simulink model "YouTubeVideo_IK_wp"  (R2023b)
settings: Solver=VariableStepAuto  StartTime=0.0  StopTime=6  RelTol=1e-3
values from neighbouring files (symbols this model uses):
  m = d(6)*ay-py    [niyundongxue.m]
undefined symbols (not defined in the file or in its folder): a1, a2, a3, d1, d4, fc1, fc2, fc3, fc4, fc5, fc6, fv1, fv2, fv3, fv4, fv5, fv6, Ia1, Ia2, Ia3, Ia4, Ia5, Ia6, Ic111, Ic112, Ic113, Ic122, Ic123, Ic133, Ic211, Ic212, Ic213, Ic222, Ic223, Ic233, Ic311, Ic312, Ic313, Ic322, Ic323, Ic333, Ic411, Ic412, Ic413, Ic422, Ic423, Ic433, Ic511, Ic512, Ic513, Ic522, Ic523, Ic533, Ic611, Ic612, Ic613, Ic622, Ic623, Ic633, Levenberg ... (+28)
libraries: sm_lib x56, nesl_utility x31, robotcorelib x3, robotmaniplib x2, simulink x2
(part 2 of 2)

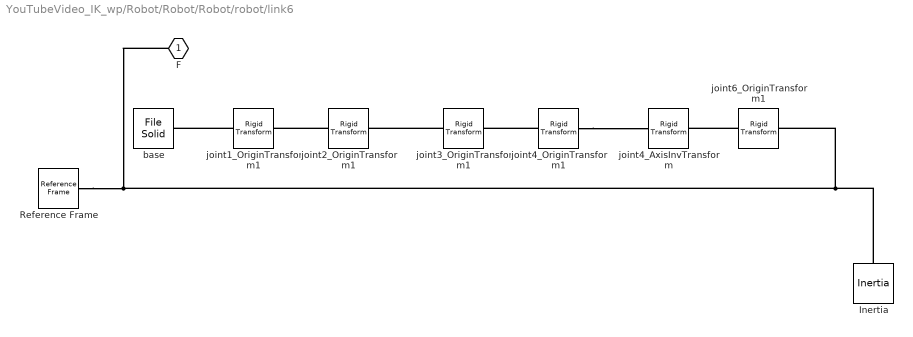
== system YouTubeVideo_IK_wp/Robot/Robot/Robot/robot/link6 ==
  Inertia : sm_lib/Body Elements/Inertia  InertiaType=Custom  Mass=m6  MassUnits=kg  CenterOfMass=[mc61 mc62 mc63]  CenterOfMassUnits=m  MomentsOfInertia=[Ic611 Ic622 Ic633 ]  MomentsOfInertiaUnits=kg*m^2  ProductsOfInertia=[Ic623 Ic613 Ic612]  ProductsOfInertiaUnits=kg*m^2  GraphicType=Marker  MarkerShape=Inertia  MarkerSize=20  GraphicVisPropType=SimpleVisualProperties  GraphicDiffuseColor=[0.5 0.5 0.5]  GraphicSpecularColor=[0.5 0.5 0.5 1.0]  GraphicAmbientColor=[0.15 0.15 0.15 1.0]  GraphicEmissiveColor=[0.0 0.0 0.0 1.0]  GraphicShininess=75  GraphicOpacity=1.0
  Reference Frame : sm_lib/Frames and Transforms/Reference Frame
  base : sm_lib/Body Elements/File Solid  ExtGeomFileName=/home/jiehuang/Documents/Custom-Robot/Matlab_Study/Matlab2023Project/IntroductionBook/程序/XB4模型/XB4-6.STL  UnitType=Custom  ExtGeomFileUnits=mm  StepReaderType=HEX  ExportConvexHullGeometry=off  InertiaType=Custom  Mass=0  MassUnits=kg  CenterOfMass=[0 0 0]  CenterOfMassUnits=m  MomentsOfInertia=[0 0 0]  MomentsOfInertiaUnits=kg*m^2  ProductsOfInertia=[0 0 0]  ProductsOfInertiaUnits=kg*m^2  BasedOnType=Density  Density=1000  DensityUnits=kg/(m^3)  DoExposeReferenceFrame=on  SerializedFrames=<Frames/>  GraphicType=FromGeometry  MarkerShape=Sphere  MarkerSize=10  GraphicVisPropType=SimpleVisualProperties  GraphicDiffuseColor=[0.5 0.5 0.5]  GraphicSpecularColor=[0.5 0.5 0.5 1.0]  GraphicAmbientColor=[0.15 0.15 0.15 1.0]  GraphicEmissiveColor=[0.0 0.0 0.0 1.0]  GraphicShininess=75  GraphicOpacity=1.0
  joint1_OriginTransform1 : sm_lib/Frames and Transforms/Rigid Transform  TranslationMethod=Cartesian  TranslationStandardOffset=0  TranslationStandardOffsetUnits=m  TranslationStandardAxis=+Z  TranslationCartesianOffset=[0 0 d1]  TranslationCartesianOffsetUnits=m  TranslationROffset=0  TranslationROffsetUnits=m  TranslationZOffset=0  TranslationZOffsetUnits=m  TranslationThetaOffset=0  TranslationThetaOffsetUnits=deg  RotationMethod=RotationSequence  RotationAngleUnits=deg  RotationStandardAxis=+Z  RotationAngle=0.0  RotationArbitraryAxis=[0 0 1]  FollAlignAxisA=+X  BaseAlignAxisA=+Y  FollAlignAxisB=+Y  BaseAlignAxisB=+Z  RotationSequenceAxes=BaseAxes  RotationSequence=XYZ  RotationSequenceAngles=[0 0 0]  RotationSequenceAnglesUnits=rad  RotationMatrix=[1 0 0; 0 1 0; 0 0 1]  Quaternion=[1 0 0 0]
  joint2_OriginTransform1 : sm_lib/Frames and Transforms/Rigid Transform  TranslationMethod=Cartesian  TranslationStandardOffset=0  TranslationStandardOffsetUnits=m  TranslationStandardAxis=+Z  TranslationCartesianOffset=[a1 0 0]  TranslationCartesianOffsetUnits=m  TranslationROffset=0  TranslationROffsetUnits=m  TranslationZOffset=0  TranslationZOffsetUnits=m  TranslationThetaOffset=0  TranslationThetaOffsetUnits=deg  RotationMethod=RotationSequence  RotationAngleUnits=deg  RotationStandardAxis=+Z  RotationAngle=0.0  RotationArbitraryAxis=[0 0 1]  FollAlignAxisA=+X  BaseAlignAxisA=+Y  FollAlignAxisB=+Y  BaseAlignAxisB=+Z  RotationSequenceAxes=FollowerAxes  RotationSequence=XYZ  RotationSequenceAngles=[-pi/2 0 -pi/2]  RotationSequenceAnglesUnits=rad  RotationMatrix=[1 0 0; 0 1 0; 0 0 1]  Quaternion=[1 0 0 0]
  joint3_OriginTransform1 : sm_lib/Frames and Transforms/Rigid Transform  TranslationMethod=Cartesian  TranslationStandardOffset=0  TranslationStandardOffsetUnits=m  TranslationStandardAxis=+Z  TranslationCartesianOffset=[a2 0 0]  TranslationCartesianOffsetUnits=m  TranslationROffset=0  TranslationROffsetUnits=m  TranslationZOffset=0  TranslationZOffsetUnits=m  TranslationThetaOffset=0  TranslationThetaOffsetUnits=deg  RotationMethod=RotationSequence  RotationAngleUnits=deg  RotationStandardAxis=+Z  RotationAngle=0.0  RotationArbitraryAxis=[0 0 1]  FollAlignAxisA=+X  BaseAlignAxisA=+Y  FollAlignAxisB=+Y  BaseAlignAxisB=+Z  RotationSequenceAxes=FollowerAxes  RotationSequence=XYZ  RotationSequenceAngles=[0 0 0]  RotationSequenceAnglesUnits=rad  RotationMatrix=[1 0 0; 0 1 0; 0 0 1]  Quaternion=[1 0 0 0]
  joint4_AxisInvTransform : sm_lib/Frames and Transforms/Rigid Transform  TranslationMethod=Cartesian  TranslationStandardOffset=0  TranslationStandardOffsetUnits=m  TranslationStandardAxis=+Z  TranslationCartesianOffset=[0 0 0]  TranslationCartesianOffsetUnits=m  TranslationROffset=0  TranslationROffsetUnits=m  TranslationZOffset=0  TranslationZOffsetUnits=m  TranslationThetaOffset=0  TranslationThetaOffsetUnits=deg  RotationMethod=RotationSequence  RotationAngleUnits=rad  RotationStandardAxis=+Z  RotationAngle=1.570796  RotationArbitraryAxis=[0 1 0]  FollAlignAxisA=+X  BaseAlignAxisA=+Y  FollAlignAxisB=+Y  BaseAlignAxisB=+Z  RotationSequenceAxes=FollowerAxes  RotationSequence=XYZ  RotationSequenceAngles=[pi/2 0 0]  RotationSequenceAnglesUnits=rad  RotationMatrix=[1 0 0; 0 1 0; 0 0 1]  Quaternion=[1 0 0 0]
  joint4_OriginTransform1 : sm_lib/Frames and Transforms/Rigid Transform  TranslationMethod=Cartesian  TranslationStandardOffset=0  TranslationStandardOffsetUnits=m  TranslationStandardAxis=+Z  TranslationCartesianOffset=[a3 d4 0]  TranslationCartesianOffsetUnits=m  TranslationROffset=0  TranslationROffsetUnits=m  TranslationZOffset=0  TranslationZOffsetUnits=m  TranslationThetaOffset=0  TranslationThetaOffsetUnits=deg  RotationMethod=RotationSequence  RotationAngleUnits=deg  RotationStandardAxis=+Z  RotationAngle=0.0  RotationArbitraryAxis=[0 0 1]  FollAlignAxisA=+X  BaseAlignAxisA=+Y  FollAlignAxisB=+Y  BaseAlignAxisB=+Z  RotationSequenceAxes=FollowerAxes  RotationSequence=XYZ  RotationSequenceAngles=[-pi/2 0 0]  RotationSequenceAnglesUnits=rad  RotationMatrix=[1 0 0; 0 1 0; 0 0 1]  Quaternion=[1 0 0 0]
  joint6_OriginTransform1 : sm_lib/Frames and Transforms/Rigid Transform  TranslationMethod=Cartesian  TranslationStandardOffset=0  TranslationStandardOffsetUnits=m  TranslationStandardAxis=+Z  TranslationCartesianOffset=[0 0 0]  TranslationCartesianOffsetUnits=m  TranslationROffset=0  TranslationROffsetUnits=m  TranslationZOffset=0  TranslationZOffsetUnits=m  TranslationThetaOffset=0  TranslationThetaOffsetUnits=deg  RotationMethod=RotationSequence  RotationAngleUnits=deg  RotationStandardAxis=+Z  RotationAngle=0.0  RotationArbitraryAxis=[0 0 1]  FollAlignAxisA=+X  BaseAlignAxisA=+Y  FollAlignAxisB=+Y  BaseAlignAxisB=+Z  RotationSequenceAxes=FollowerAxes  RotationSequence=XYZ  RotationSequenceAngles=[-pi/2 0 0]  RotationSequenceAnglesUnits=rad  RotationMatrix=[1 0 0; 0 1 0; 0 0 1]  Quaternion=[1 0 0 0]
  F : PMIOPort  Side=Left
  connections:
  Reference Frame/RConn1 -- joint6_OriginTransform1/RConn1 -- Inertia/RConn1 -- F/RConn1
  joint6_OriginTransform1/LConn1 -- joint4_AxisInvTransform/RConn1
  joint1_OriginTransform1/LConn1 -- base/RConn1
  joint3_OriginTransform1/LConn1 -- joint2_OriginTransform1/RConn1
  joint4_OriginTransform1/RConn1 -- joint4_AxisInvTransform/LConn1
  joint4_OriginTransform1/LConn1 -- joint3_OriginTransform1/RConn1
  joint2_OriginTransform1/LConn1 -- joint1_OriginTransform1/RConn1

== matlab function YouTubeVideo_IK_wp/Robot/Robot/Robot/robot/friction ==
  data: u input; y output; fv input; fc input
function y = fcn(u,fv,fc)
%#codegen


% fv1=100; fc1=80; fv2=150; fc2=100; fv3=100; fc3=50; fv4=80; fc4=80; fv5=50; fc5=30; fv6=30; fc6=10;
fv1=fv(1); fc1=fc(1); fv2=fv(2); fc2=fc(2); fv3=fv(3); fc3=fc(3); fv4=fv(4); fc4=fc(4); fv5=fv(5); fc5=fc(5); fv6=fv(6); fc6=fc(6);
y=[0;0;0;0;0;0];
y(1)=(fv1*u(1)+fc1*sign(u(1)));
y(2)=(fv2*u(2)+fc2*sign(u(2)));
y(3)=(fv3*u(3)+fc3*sign(u(3)));
y(4)=(fv4*u(4)+fc4*sign(u(4)));
y(5)=(fv5*u(5)+fc5*sign(u(5)));
y(6)=(fv6*u(6)+fc6*sign(u(6)));

end

== matlab function YouTubeVideo_IK_wp/Robot/Robot/Robot/robot/Jm ==
  data: u input; y output; Jm input
function y = fcn(u,Jm)
%#codegen

% Jm=[200; 250; 150; 100; 50; 20];%关节惯性
y = Jm.*u;
end
